simulink subsystem "Sensor"  (R2023b)
settings: Solver=VariableStepAuto  StartTime=0.0  StopTime=10.0  RelTol=1e-3
libraries: arduinolib x2
settings Model: Creator=chaya  LastModifiedBy=chaya

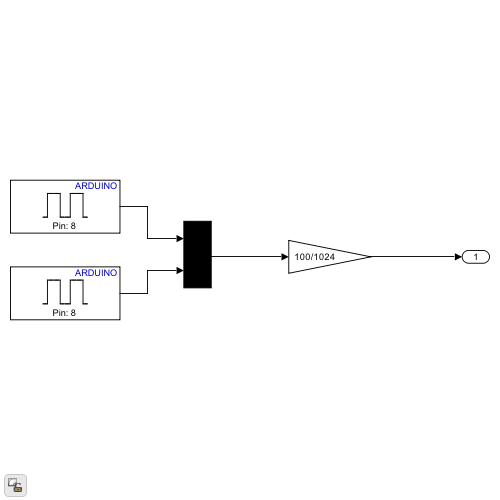
[thumbnail: Simulink's stored preview of the top-level diagram]
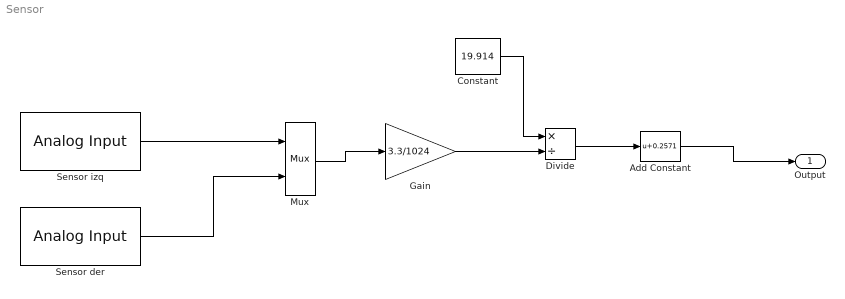
== system Sensor ==
  Add Constant : Bias  Bias=0.2571  SaturateOnIntegerOverflow=off
  Constant : Constant  Value=19.914
  Divide : Product  Inputs=*/
  Gain : Gain  Gain=3.3/1024
  Mux : Mux  Inputs=2
  Sensor der : arduinolib/Analog Input  pinNumber=0  ReadResultsOnly=off  ConversionTriggerSource=Software  ExternalTriggerType=uint32( 0 )  OutputDataType=uint16  EnableConversionCompleteNotify=off  EnableOuputStatus=off  SampleTime=-1  blockPlatform=arduino
  Sensor izq : arduinolib/Analog Input  pinNumber=1  ReadResultsOnly=off  ConversionTriggerSource=Software  ExternalTriggerType=uint32( 0 )  OutputDataType=uint16  EnableConversionCompleteNotify=off  EnableOuputStatus=off  SampleTime=-1  blockPlatform=arduino
  Output : Outport
  wires:
  Sensor izq/1 -> Mux/1
  Sensor der/1 -> Mux/2
  Gain/1 -> Divide/2
  Constant/1 -> Divide/1
  Divide/1 -> Add Constant/1
  Add Constant/1 -> Output/1
  Mux/1 -> Gain/1
